simulink model "test_for_orbital_evolution"  (R2024a)
settings: Solver=VariableStepAuto  StartTime=0.0  StopTime=120  RelTol=1e-3
values from neighbouring files (symbols this model uses):
  e_orbit = 0    [Initiate_FQ.m]
  e_orbit_t = (mu_orbit_t^2/mu_earth)/radius_orbit_t-1    [Initiate_FQ.m]
  Mean_Anomaly0 = MeanAnomaly(e_orbit,E0)    [Initiate_FQ.m]
  Mean_Anomaly0_t = MeanAnomaly(e_orbit,E0)    [Initiate_FQ.m]
  mu_earth = 3.986004418*10^14    (= 398600441800000)    [Initiate_FQ.m]
  mu_orbit = sqrt(radius_orbit*mu_earth)    [Initiate_FQ.m]
  mu_orbit_t = radius_orbit_t*vel_orbit_t    [Initiate_FQ.m]
  n_orbit = (mu_earth^2)/(mu_orbit^3)    [Initiate_FQ.m]
  n_orbit_t = (mu_earth^2)/(mu_orbit^3)    [Initiate_FQ.m]
  theta0 = 0    [Initiate_FQ.m]
  theta0_t = 0    [Initiate_FQ.m]
settings Model: Creator=Bmmog  LastModifiedBy=Bmmog

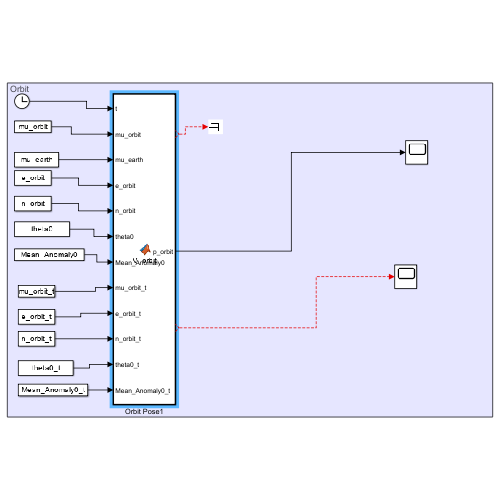
[thumbnail: Simulink's stored preview of the top-level diagram]
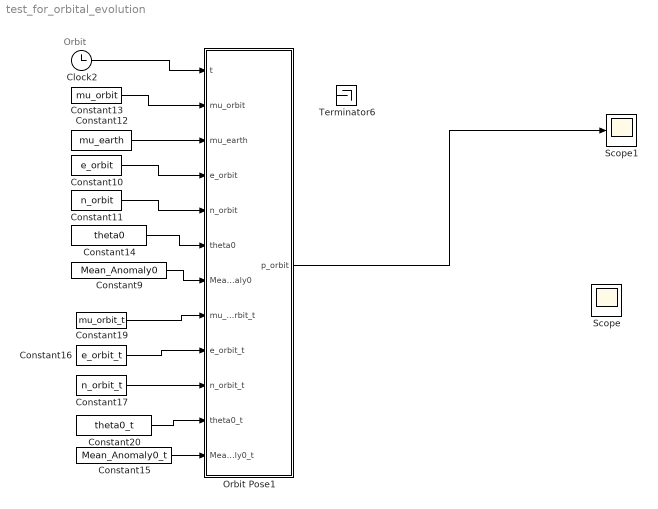
== system test_for_orbital_evolution ==
  note: Orbit
  Clock2 : Clock
  Constant10 : Constant  Value=e_orbit
  Constant11 : Constant  Value=n_orbit
  Constant12 : Constant  Value=mu_earth
  Constant13 : Constant  Value=mu_orbit
  Constant14 : Constant  Value=theta0
  Constant15 : Constant  Value=Mean_Anomaly0_t
  Constant16 : Constant  Value=e_orbit_t
  Constant17 : Constant  Value=n_orbit_t
  Constant19 : Constant  Value=mu_orbit_t
  Constant20 : Constant  Value=theta0_t
  Constant9 : Constant  Value=Mean_Anomaly0
  Orbit Pose1 : MATLAB Function  TreatAsAtomicUnit=on
  Scope : Scope
  Scope1 : Scope
  Terminator6 : Terminator
  wires:
  Clock2/1 -> Orbit Pose1/1(t)
  Constant19/1 -> Orbit Pose1/8(mu_orbit_t)
  Constant20/1 -> Orbit Pose1/11(theta0_t)
  Constant12/1 -> Orbit Pose1/3(mu_earth)
  Constant16/1 -> Orbit Pose1/9(e_orbit_t)
  Constant15/1 -> Orbit Pose1/12(Mean_Anomaly0_t)
  ? -> Terminator6/1
  Constant9/1 -> Orbit Pose1/7(Mean_Anomaly0)
  Constant11/1 -> Orbit Pose1/5(n_orbit)
  Constant14/1 -> Orbit Pose1/6(theta0)
  Constant13/1 -> Orbit Pose1/2(mu_orbit)
  Constant17/1 -> Orbit Pose1/10(n_orbit_t)
  Constant10/1 -> Orbit Pose1/4(e_orbit)
  Orbit Pose1/1(p_orbit) -> Scope1/1
  ? -> Scope/1

== matlab function test_for_orbital_evolution/Orbit Pose1 ==
  data: t input; mu_orbit input; mu_earth input; e_orbit input; n_orbit input; theta0 input; Mean_Anomaly0 input; p_orbit output; mu_orbit_t input; e_orbit_t input; n_orbit_t input; theta0_t input; Mean_Anomaly0_t input
function p_orbit  = V_orbit(t,mu_orbit, mu_earth, e_orbit,n_orbit,theta0, Mean_Anomaly0, mu_orbit_t, e_orbit_t,n_orbit_t,theta0_t, Mean_Anomaly0_t)

theta=find_theta(t,e_orbit,n_orbit,Mean_Anomaly0);

%E=0.5*MA_inv( Mean_Anomaly0 + (P_orb^(3/2)/mu_earth*t ));
%theta=2*atan(   ((1-e)/(1+e)) *tan(E));
%theta0=0;

%p_orbit=(mu_orbit^2/mu_earth)*[1/(1+e*cos(theta))-(cos(theta-theta0))/(1+e*cos(theta0)); (sin(theta-theta0))/(1+e*cos(theta0));   0];
% V_inertia_curly=(mu_earth/mu_orbit)*[-sin(theta0); e_orbit+cos(theta0);    0];
% 
% V_inertia=V_inertia_curly;

%p_orbit=(mu_orbit^2/mu_earth)*[1/(1+e*cos(theta))-(cos(theta-theta0))/(1+e*cos(theta0)); (sin(theta-theta0))/(1+e*cos(theta0));   0];
p_orbit=(mu_orbit^2/mu_earth)/(1+e_orbit*cos(theta))*([cos(theta);sin(theta);0]);%-[cos(theta0);sin(theta0);0])-V_inertia*t;
% R_orbit=[cos(theta-theta0) sin(theta-theta0) 0; -sin(theta-theta0) cos(theta-theta0) 0; 0 0 1];

% theta_z=theta-theta0;
% w_z=(mu_earth)^2/(mu_orbit^3)*(1+e_orbit*cos(theta))^2;

%-------------------------------------------

theta_t=find_theta(t,e_orbit_t,n_orbit_t,Mean_Anomaly0_t);

%E=0.5*MA_inv( Mean_Anomaly0 + (P_orb^(3/2)/mu_earth*t ));
%theta=2*atan(   ((1-e)/(1+e)) *tan(E));
%theta0=0;

%p_orbit=(mu_orbit^2/mu_earth)*[1/(1+e*cos(theta))-(cos(theta-theta0))/(1+e*cos(theta0)); (sin(theta-theta0))/(1+e*cos(theta0));   0];
% V_inertia_curly_t=(mu_earth/mu_orbit_t)*[-sin(theta0_t); e_orbit_t+cos(theta0_t);    0];
% 
% V_inertia_t=V_inertia_curly_t;

%p_orbit=(mu_orbit^2/mu_earth)*[1/(1+e*cos(theta))-(cos(theta-theta0))/(1+e*cos(theta0)); (sin(theta-theta0))/(1+e*cos(theta0));   0];
p_orbit_t=(mu_orbit_t^2/mu_earth)/(1+e_orbit_t*cos(theta_t))*([cos(theta_t);sin(theta_t);0]);%-[cos(theta0_t);sin(theta0_t);0])-V_inertia_t*t;
% R_orbit_t=[cos(theta_t-theta0_t) sin(theta_t-theta0_t) 0; -sin(theta_t-theta0_t) cos(theta_t-theta0_t) 0; 0 0 1];

% theta_z_t=theta_t-theta0_t;
% w_z_t=(mu_earth)^2/(mu_orbit_t^3)*(1+e_orbit_t*cos(theta_t))^2;

p_orbit=p_orbit-p_orbit_t;
% theta_z=theta_z-theta_z_t;
